simulink model "TestDrag"  (R2015a)
settings: Solver=ode45  StartTime=0.0  StopTime=inf  FixedStep=0.01  RelTol=1e-3
libraries: dspindex x9, simulink x7, dspnetwork x3, aerolibconvert2 x2, IMU_Library x1, GPS_Library x1, realtime_pacer_lib x1, etargetslib x1
settings Model: ParamWorkspaceSource=ReferencedWorkspace  CovSFcnEnable=off  Creator=abdkadma  LastModifiedBy=theth
settings OptimizationCC: InlineParams=on  InlineInvariantSignals=on  EnhancedBackFolding=on  ExpressionDepthLimit=2147483647  EfficientFloat2IntCast=on  SimCompilerOptimization=on
settings DebuggingCC: UnderspecifiedInitializationDetection=Classic  MergeDetectMultiDrivingBlocksExec=none  SolverPrmCheckMsg=warning  StateNameClashWarn=warning
settings RTWCC: RTWCompilerOptimization=on  CheckMdlBeforeBuild=Warning
settings GRTTargetCC: MatFileLogging=off  SupportNonFinite=off

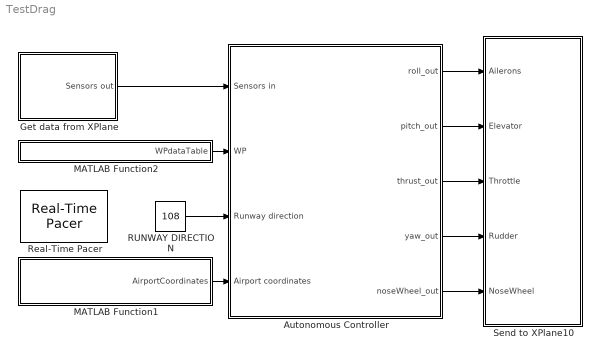
== system TestDrag ==
  "Autonomous Controller " : Subsystem
  Get data from XPlane : Subsystem  Description=|  TreatAsAtomicUnit=on  mask(Get Data from Xplane10){remoteURL='127.0.0.1', localPort=49005, sampletime=0.02}
      | Done by: Mohamed Abdelkader
      | Contact for updates: mohamedashraf123@gmail.com
      mask prompts: remoteURL "Remote IP address ('0.0.0.0' to accept all):(default='127.0.0.1')"; localPort "Local IP port: that Xplane10 sends to (default=49005)"; sampletime "Sampling time (seconds), how frequenlty to capture data from Xplane. Don't set to low as it might not be able to capture the smaples from Xplane. Default is 0.02 assuming the UDP rate in Xplane is set to 50 sample per second"
      mask help:
      | Get Data from X-Plane10
      | * make sure you configure the right port
      | and the right IP address
      mask TypeOptions remoteURL: UDP Receive1/remoteURL
      mask TypeOptions localPort: UDP Receive1/localPort
      mask TypeOptions sampletime: UDP Receive1/sampletime
  MATLAB Function1 : MATLAB Function  TreatAsAtomicUnit=on
  MATLAB Function2 : MATLAB Function  TreatAsAtomicUnit=on
  RUNWAY DIRECTION : Constant  Value=108
  Real-Time Pacer : realtime_pacer_lib/Real-Time Pacer  simTimePerRealTime=1
  Send to XPlane10 : Subsystem  Description=|  mask(Send Commands to X-Plane 10){remoteURL='127.0.0.1', remotePort=49000}
      | Done by: Mohamed Abdelkader
      | Contact for updates: mohamedashraf123@gmail.com
      mask prompts: remoteURL "Remote IP address (default='127.0.0.1'): X-Plane10 IP"; remotePort "Remote IP port:X-Plane10 port(default=49000)"
      mask help:
      | Sends Control Surfaces Commands to Xplane10
      | Throttle in [0,1]
      | Elevator, Ailerons, rudder, nosewheel in [-1,1]
      mask TypeOptions remoteURL: UDP Send/remoteURL
      mask TypeOptions remotePort: UDP Send/remotePort
  wires:
  "Autonomous Controller "/1(roll_out) -> Send to XPlane10/1(Ailerons)
  "Autonomous Controller "/2(pitch_out) -> Send to XPlane10/2(Elevator)
  "Autonomous Controller "/3(thrust_out) -> Send to XPlane10/3(Throttle)
  "Autonomous Controller "/4(yaw_out) -> Send to XPlane10/4(Rudder)
  "Autonomous Controller "/5(noseWheel_out) -> Send to XPlane10/5(NoseWheel)
  Get data from XPlane/1(Sensors out) -> "Autonomous Controller "/1(Sensors in)
  RUNWAY DIRECTION/1 -> "Autonomous Controller "/3(Runway direction)
  MATLAB Function1/1(AirportCoordinates) -> "Autonomous Controller "/4(Airport coordinates)
  MATLAB Function2/1(WPdataTable) -> "Autonomous Controller "/2(WP)

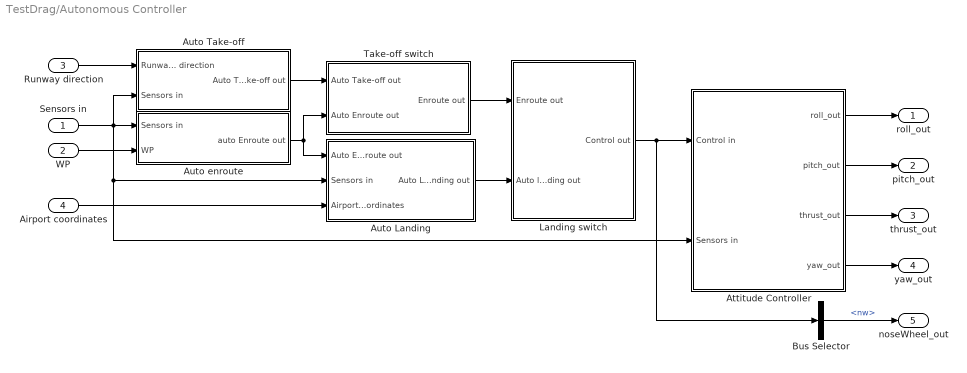
== system TestDrag/Autonomous Controller  ==
  Sensors in : Inport
  WP : Inport  Port=2
  Runway direction : Inport  Port=3
  Airport coordinates : Inport  Port=4
  Attitude Controller : Subsystem
  Auto Landing : Subsystem
  Auto Take-off : Subsystem
  Auto enroute : Subsystem
  Bus Selector : BusSelector  OutputSignals=nw
  Landing switch : Subsystem
  Take-off switch : Subsystem
  roll_out : Outport
  pitch_out : Outport  Port=2
  thrust_out : Outport  Port=3
  yaw_out : Outport  Port=4
  noseWheel_out : Outport  Port=5
  wires:
  Take-off switch/1(Enroute out) -> Landing switch/1(Enroute out)
  Auto Landing/1(Auto Landing out) -> Landing switch/2(Auto landing out)
  Auto enroute/1(auto Enroute out) -> Auto Landing/1(Auto Enroute out), Take-off switch/2(Auto Enroute out)
  Attitude Controller/4(yaw_out) -> yaw_out/1
  Attitude Controller/1(roll_out) -> roll_out/1
  Attitude Controller/3(thrust_out) -> thrust_out/1
  Auto Take-off/1(Auto Take-off out) -> Take-off switch/1(Auto Take-off out)
  Sensors in/1 -> Auto enroute/1(Sensors in), Auto Take-off/2(Sensors in), Attitude Controller/2(Sensors in), Auto Landing/2(Sensors in)
  Runway direction/1 -> Auto Take-off/1(Runway direction)
  Landing switch/1(Control out) -> Attitude Controller/1(Control in), Bus Selector/1
  Bus Selector/1 -> noseWheel_out/1  "<nw>"
  Attitude Controller/2(pitch_out) -> pitch_out/1
  Airport coordinates/1 -> Auto Landing/3(Airport coordinates)
  WP/1 -> Auto enroute/2(WP)

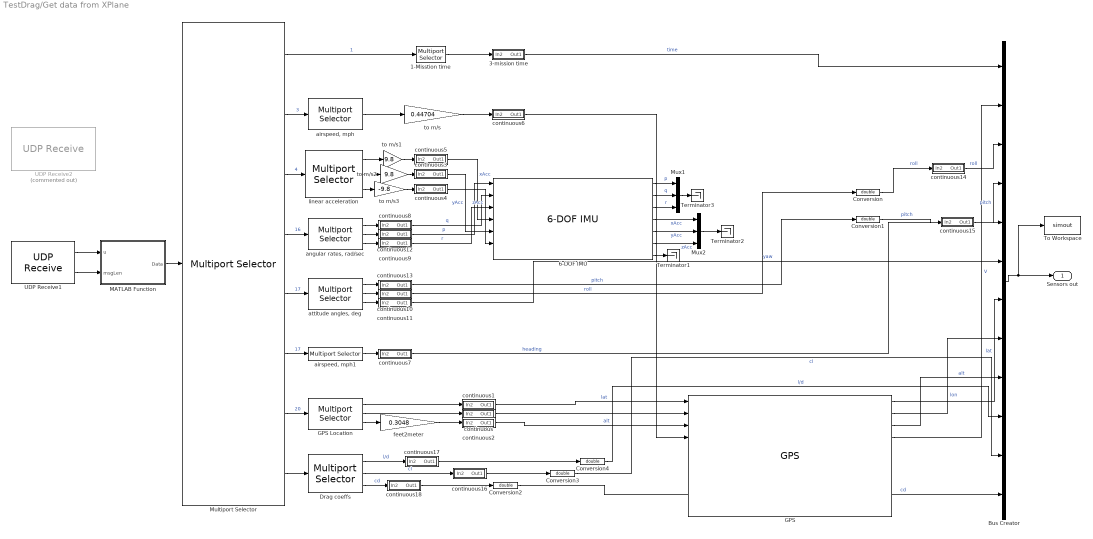
== system TestDrag/Get data from XPlane ==
  1-Misstion time : dspindex/Multiport Selector  rowsOrCols=Columns  idxCellArray={3}  idxErrMode=Clip Index
  3-mission time : Subsystem
  6-DOF IMU : IMU_Library/6-DOF IMU  lpf_filt_freq_hz_ix=20 Hz  gyro_scale_ix=+/- 500 deg/sec  accel_scale_ix=+/- 8g  SampleTime=0.02  lpf_filt_freq_hz=5 Hz  gyro_scale=+/- 250 deg/sec  accel_scale=+/- 2g
  Bus Creator : BusCreator  Inputs='time','V','roll','pitch','heading','yaw','lat','lon','alt','l/d','cl','cd'
  Conversion{,1..4} (5 alike) : DataTypeConversion  OutDataTypeStr=double
  Drag coeffs : dspindex/Multiport Selector  rowsOrCols=Columns  idxCellArray={1,3,4}  idxErrMode=Clip Index
  GPS : GPS_Library/GPS
  GPS Location : dspindex/Multiport Selector  rowsOrCols=Columns  idxCellArray={1,2,3}  idxErrMode=Clip Index
  MATLAB Function : MATLAB Function  TreatAsAtomicUnit=on
  Multiport Selector : dspindex/Multiport Selector  rowsOrCols=Rows  idxCellArray={1,3,4,16,17,18,20,68}  idxErrMode=Clip Index
  Mux1 : Mux  Inputs=3
  Mux2 : Mux  Inputs=3
  Terminator1 : Terminator
  Terminator2 : Terminator
  Terminator3 : Terminator
  To Workspace : ToWorkspace  VariableName=simout  SampleTime=-1
      settings: Save2DSignal=2-D array (concatenate along first dimension)
  UDP Receive1 : dspnetwork/UDP Receive  localURL='0.0.0.0'  localPort=localPort  remoteURL=remoteURL  remotePort=-1  recvBufferSize=8192  dims=365*20  signalDatatype=uint8  isVarSize=off  showBlockingTime=off  blockingTime=0  sampletime=sampletime
  UDP Receive2 : dspnetwork/UDP Receive  Commented=on  localURL='0.0.0.0'  localPort=localPort  remoteURL=remoteURL  remotePort=-1  recvBufferSize=8192  dims=365  signalDatatype=uint8  isVarSize=off  showBlockingTime=on  blockingTime=0.01  sampletime=0.01  blockPlatform=LINUX
  "airspeed, mph" : dspindex/Multiport Selector  rowsOrCols=Columns  idxCellArray={6}  idxErrMode=Clip Index
  "airspeed, mph1" : dspindex/Multiport Selector  rowsOrCols=Columns  idxCellArray={3}  idxErrMode=Clip Index
  "angular rates, rad/sec" : dspindex/Multiport Selector  rowsOrCols=Columns  idxCellArray={1,2,3}  idxErrMode=Clip Index
  "attitude angles, deg" : dspindex/Multiport Selector  rowsOrCols=Columns  idxCellArray={1,2,3}  idxErrMode=Clip Index
  continuous : Subsystem
  continuous1 : Subsystem
  continuous10 : Subsystem
  continuous11 : Subsystem
  continuous12 : Subsystem
  continuous13 : Subsystem
  continuous14 : Subsystem
  continuous15 : Subsystem
  continuous16 : Subsystem
  continuous17 : Subsystem
  continuous18 : Subsystem
  continuous2 : Subsystem
  continuous3 : Subsystem
  continuous4 : Subsystem
  continuous5 : Subsystem
  continuous6 : Subsystem
  continuous7 : Subsystem
  continuous8 : Subsystem
  continuous9 : Subsystem
  feet2meter : Gain  Gain=0.3048
  linear acceleration : dspindex/Multiport Selector  rowsOrCols=Columns  idxCellArray={6,7,5}  idxErrMode=Clip Index
  to m/s : Gain  Gain=0.44704
  to m/s1 : Gain  Gain=9.8
  to m/s2 : Gain  Gain=9.8
  to m/s3 : Gain  Gain=-9.8
  Sensors out : Outport
  wires:
  "attitude angles, deg"/3 -> continuous11/1(In2)
  "angular rates, rad/sec"/3 -> continuous9/1(In2)
  MATLAB Function/1(Data) -> Multiport Selector/1
  linear acceleration/2 -> to m/s2/1
  to m/s2/1 -> continuous3/1(In2)
  to m/s1/1 -> continuous5/1(In2)
  "attitude angles, deg"/1 -> continuous13/1(In2)
  "attitude angles, deg"/2 -> continuous10/1(In2)
  to m/s/1 -> continuous6/1(In2)
  "airspeed, mph"/1 -> to m/s/1
  linear acceleration/1 -> to m/s1/1
  "angular rates, rad/sec"/1 -> continuous8/1(In2)
  linear acceleration/3 -> to m/s3/1
  "angular rates, rad/sec"/2 -> continuous12/1(In2)
  "airspeed, mph1"/1 -> continuous7/1(In2)
  to m/s3/1 -> continuous4/1(In2)
  feet2meter/1 -> continuous2/1(In2)
  UDP Receive1/1 -> MATLAB Function/1(u)
  UDP Receive1/2 -> MATLAB Function/2(msgLen)
  GPS Location/3 -> feet2meter/1
  GPS Location/2 -> continuous/1(In2)
  GPS Location/1 -> continuous1/1(In2)
  continuous11/1(Out1) -> Bus Creator/6  "yaw"
  Bus Creator/1 -> To Workspace/1, Sensors out/1
  Multiport Selector/4 -> "angular rates, rad/sec"/1  "16"
  Multiport Selector/5 -> "attitude angles, deg"/1  "17"
  Multiport Selector/6 -> "airspeed, mph1"/1  "17"
  Multiport Selector/7 -> GPS Location/1  "20"
  1-Misstion time/1 -> 3-mission time/1(In2)
  Multiport Selector/1 -> 1-Misstion time/1  "1"
  Multiport Selector/2 -> "airspeed, mph"/1  "3"
  Multiport Selector/3 -> linear acceleration/1  "4"
  continuous5/1(Out1) -> 6-DOF IMU/4  "xAcc"
  continuous3/1(Out1) -> 6-DOF IMU/5  "yAcc"
  continuous4/1(Out1) -> 6-DOF IMU/6  "zAcc"
  continuous12/1(Out1) -> 6-DOF IMU/1  "p"
  continuous8/1(Out1) -> 6-DOF IMU/2  "q"
  continuous9/1(Out1) -> 6-DOF IMU/3  "r"
  continuous1/1(Out1) -> GPS/1  "lat"
  GPS/1 -> Bus Creator/7  "lat"
  continuous/1(Out1) -> GPS/2
  GPS/2 -> Bus Creator/8  "lon"
  continuous2/1(Out1) -> GPS/3  "alt"
  GPS/3 -> Bus Creator/9  "alt"
  continuous6/1(Out1) -> GPS/4
  GPS/4 -> Bus Creator/2  "V"
  continuous7/1(Out1) -> Bus Creator/5  "heading"
  3-mission time/1(Out1) -> Bus Creator/1  "time"
  6-DOF IMU/7 -> Terminator1/1
  6-DOF IMU/1 -> Mux1/1  "p"
  6-DOF IMU/2 -> Mux1/2  "q"
  6-DOF IMU/3 -> Mux1/3  "r"
  6-DOF IMU/4 -> Mux2/1  "xAcc"
  6-DOF IMU/5 -> Mux2/2  "yAcc"
  6-DOF IMU/6 -> Mux2/3  "zAcc"
  continuous13/1(Out1) -> Conversion1/1  "pitch"
  continuous10/1(Out1) -> Conversion/1  "roll"
  Conversion/1 -> continuous14/1(In2)  "roll"
  Conversion1/1 -> continuous15/1(In2)  "pitch"
  continuous14/1(Out1) -> Bus Creator/3  "roll"
  continuous15/1(Out1) -> Bus Creator/4  "pitch"
  Mux1/1 -> Terminator3/1
  Mux2/1 -> Terminator2/1
  Multiport Selector/8 -> Drag coeffs/1
  Drag coeffs/1 -> continuous17/1(In2)  "l/d"
  Drag coeffs/2 -> continuous16/1(In2)  "cl"
  Drag coeffs/3 -> continuous18/1(In2)  "cd"
  Conversion2/1 -> Bus Creator/12  "cd"
  Conversion3/1 -> Bus Creator/11  "cl"
  Conversion4/1 -> Bus Creator/10  "l/d"
  continuous17/1(Out1) -> Conversion4/1
  continuous16/1(Out1) -> Conversion3/1
  continuous18/1(Out1) -> Conversion2/1

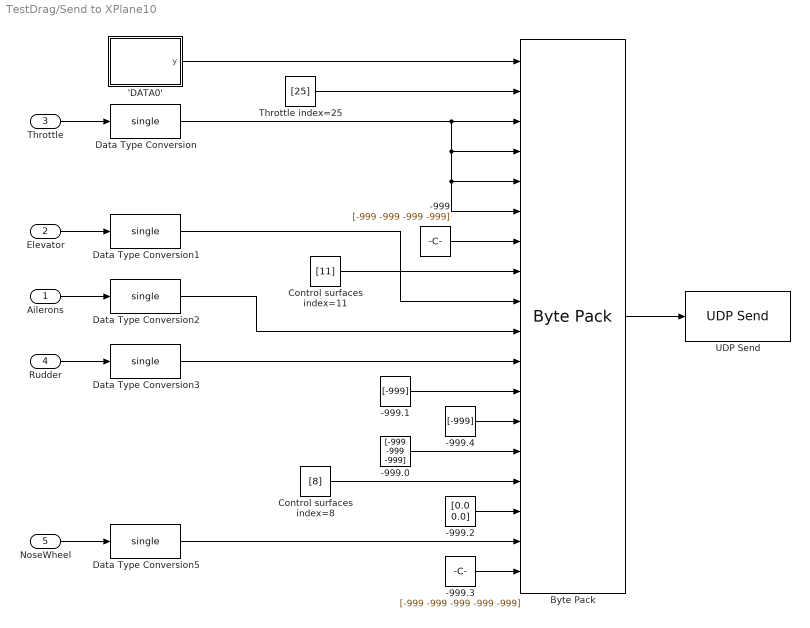
== system TestDrag/Send to XPlane10 ==
  Ailerons : Inport
  Elevator : Inport  Port=2
  Throttle : Inport  Port=3
  Rudder : Inport  Port=4
  NoseWheel : Inport  Port=5
  'DATA0' : MATLAB Function  TreatAsAtomicUnit=on
  -999 : Constant  Value=[-999 -999 -999 -999]  OutDataTypeStr=int32  SampleTime=-1
  -999.0 : Constant  Value=[-999 -999 -999]  OutDataTypeStr=int32  SampleTime=-1
  -999.1 : Constant  Value=[-999]  OutDataTypeStr=int32  SampleTime=-1
  -999.2 : Constant  Value=[0.0 0.0]  OutDataTypeStr=single  SampleTime=-1
  -999.3 : Constant  Value=[-999 -999 -999 -999 -999]  OutDataTypeStr=int32  SampleTime=-1
  -999.4 : Constant  Value=[-999]  OutDataTypeStr=single  SampleTime=-1
  Byte Pack : etargetslib/Byte Pack  datatypes={'uint8','uint32','single','single','single','single','int32','uint32','single','single','single','int32','single','int32','uint32','single','single','int32'}  byteAlign=1
  Control surfaces index=11 : Constant  Value=[11]  OutDataTypeStr=uint32  SampleTime=-1
  Control surfaces index=8 : Constant  Value=[8]  OutDataTypeStr=uint32  SampleTime=-1
  Data Type Conversion : DataTypeConversion  OutMin=[0]  OutMax=[1.0]  OutDataTypeStr=single
  Data Type Conversion{1..3,5} (4 alike) : DataTypeConversion  OutMin=[-1.0]  OutMax=[1.0]  OutDataTypeStr=single
  Throttle index=25 : Constant  Value=[25]  OutDataTypeStr=uint32  SampleTime=-1
  UDP Send : dspnetwork/UDP Send  remoteURL=remoteURL  remotePort=remotePort  localURL='0.0.0.0'  localPortSource=Automatically determine  localPort=-1  sampletime=-1  separateLengthPort=0
  wires:
  Ailerons/1 -> Data Type Conversion2/1
  Control surfaces index=11/1 -> Byte Pack/8
  Throttle/1 -> Data Type Conversion/1
  Data Type Conversion1/1 -> Byte Pack/9
  'DATA0'/1(y) -> Byte Pack/1
  Throttle index=25/1 -> Byte Pack/2
  Byte Pack/1 -> UDP Send/1
  -999/1 -> Byte Pack/7
  Data Type Conversion2/1 -> Byte Pack/10
  Data Type Conversion3/1 -> Byte Pack/11
  Rudder/1 -> Data Type Conversion3/1
  -999.0/1 -> Byte Pack/14
  Elevator/1 -> Data Type Conversion1/1
  Data Type Conversion/1 -> Byte Pack/3, Byte Pack/4, Byte Pack/6, Byte Pack/5
  -999.1/1 -> Byte Pack/12
  Control surfaces index=8/1 -> Byte Pack/15
  -999.2/1 -> Byte Pack/16
  Data Type Conversion5/1 -> Byte Pack/17
  NoseWheel/1 -> Data Type Conversion5/1
  -999.3/1 -> Byte Pack/18
  -999.4/1 -> Byte Pack/13

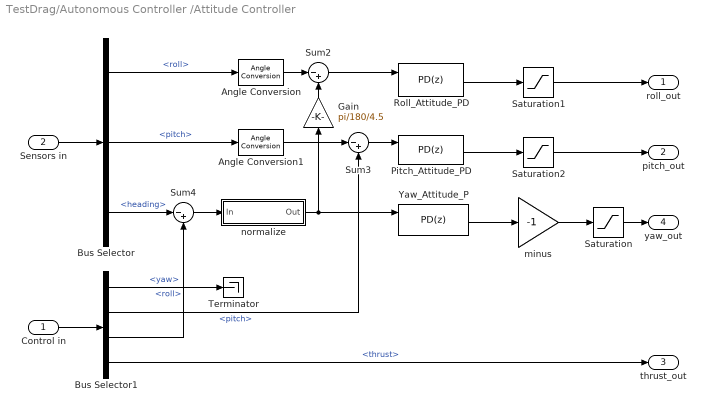
== system TestDrag/Autonomous Controller /Attitude Controller ==
  Control in : Inport
  Sensors in : Inport  Port=2
  Angle Conversion : aerolibconvert2/Angle Conversion  IU=deg  OU=rad
  Angle Conversion1 : aerolibconvert2/Angle Conversion  IU=deg  OU=rad
  Bus Selector : BusSelector  OutputSignals=roll,pitch,heading
  Bus Selector1 : BusSelector  OutputSignals=roll,pitch,yaw,thrust
  Gain : Gain  Gain=pi/180/4.5
  Pitch_Attitude_PD : simulink/Continuous/PID Controller  Controller=PD  TimeDomain=Discrete-time  SampleTime=0.02  IntegratorMethod=Forward Euler  FilterMethod=Forward Euler  Form=Parallel  UseFilter=off  ControllerParametersSource=internal  P=1  I=0  D=0.04  N=20  InitialConditionSource=internal  InitialConditionForIntegrator=0  InitialConditionForFilter=0  ExternalReset=either  LimitOutput=on  UpperSaturationLimit=1  LowerSaturationLimit=-1  LinearizeAsGain=on  AntiWindupMode=none  Kb=1  TrackingMode=off  Kt=1  PParamMin=[]  PParamMax=[]  IParamMin=[]  IParamMax=[]  DParamMin=[]  DParamMax=[]  NParamMin=[]  NParamMax=[]  KbParamMin=[]  KbParamMax=[]  KtParamMin=[]  KtParamMax=[]  POutMin=[]  POutMax=[]  IOutMin=[]  IOutMax=[]  DOutMin=[]  DOutMax=[]  NOutMin=[]  NOutMax=[]  KbOutMin=[]  KbOutMax=[]  KtOutMin=[]  KtOutMax=[]  IntegratorOutMin=[]  IntegratorOutMax=[]  FilterOutMin=[]  FilterOutMax=[]  SumOutMin=[]  SumOutMax=[]  SumI1OutMin=[]  SumI1OutMax=[]  SumI2OutMin=[]  SumI2OutMax=[]  SumI3OutMin=[]  SumI3OutMax=[]  SumDOutMin=[]  SumDOutMax=[]  SaturationOutMin=[]  SaturationOutMax=[]  IntegratorContinuousStateAttributes=''  IntegratorStateMustResolveToSignalObject=off  IntegratorRTWStateStorageClass=Auto  FilterContinuousStateAttributes=''  FilterStateMustResolveToSignalObject=off  FilterRTWStateStorageClass=Auto  DifferentiatorICPrevScaledInput=0  DifferentiatorOutMin=[]  DifferentiatorOutMax=[]
  Roll_Attitude_PD : simulink/Continuous/PID Controller  Controller=PD  TimeDomain=Discrete-time  SampleTime=0.02  IntegratorMethod=Forward Euler  FilterMethod=Forward Euler  Form=Parallel  UseFilter=off  ControllerParametersSource=internal  P=1  I=0  D=0.0008  N=20  InitialConditionSource=internal  InitialConditionForIntegrator=0  InitialConditionForFilter=0  ExternalReset=either  LimitOutput=on  UpperSaturationLimit=1  LowerSaturationLimit=-1  LinearizeAsGain=on  AntiWindupMode=none  Kb=1  TrackingMode=off  Kt=1  PParamMin=[]  PParamMax=[]  IParamMin=[]  IParamMax=[]  DParamMin=[]  DParamMax=[]  NParamMin=[]  NParamMax=[]  KbParamMin=[]  KbParamMax=[]  KtParamMin=[]  KtParamMax=[]  POutMin=[]  POutMax=[]  IOutMin=[]  IOutMax=[]  DOutMin=[]  DOutMax=[]  NOutMin=[]  NOutMax=[]  KbOutMin=[]  KbOutMax=[]  KtOutMin=[]  KtOutMax=[]  IntegratorOutMin=[]  IntegratorOutMax=[]  FilterOutMin=[]  FilterOutMax=[]  SumOutMin=[]  SumOutMax=[]  SumI1OutMin=[]  SumI1OutMax=[]  SumI2OutMin=[]  SumI2OutMax=[]  SumI3OutMin=[]  SumI3OutMax=[]  SumDOutMin=[]  SumDOutMax=[]  SaturationOutMin=[]  SaturationOutMax=[]  IntegratorContinuousStateAttributes=''  IntegratorStateMustResolveToSignalObject=off  IntegratorRTWStateStorageClass=Auto  FilterContinuousStateAttributes=''  FilterStateMustResolveToSignalObject=off  FilterRTWStateStorageClass=Auto  DifferentiatorICPrevScaledInput=0  DifferentiatorOutMin=[]  DifferentiatorOutMax=[]
  Saturation : Saturate  UpperLimit=1  LowerLimit=-1
  Saturation1 : Saturate  UpperLimit=0.05  LowerLimit=-0.05
  Saturation2 : Saturate  UpperLimit=1  LowerLimit=-1
  Sum2 : Sum  Inputs=|-+
  Sum3 : Sum  Inputs=|-+
  Sum4 : Sum  Inputs=|-+
  Terminator : Terminator
  Yaw_Attitude_P : simulink/Continuous/PID Controller  Controller=PD  TimeDomain=Discrete-time  SampleTime=0.02  IntegratorMethod=Forward Euler  FilterMethod=Forward Euler  Form=Parallel  UseFilter=off  ControllerParametersSource=internal  P=pi/180  I=0  D=0.000034  N=100  InitialConditionSource=internal  InitialConditionForIntegrator=0  InitialConditionForFilter=0  ExternalReset=either  LimitOutput=on  UpperSaturationLimit=1  LowerSaturationLimit=-1  LinearizeAsGain=on  AntiWindupMode=none  Kb=1  TrackingMode=off  Kt=1  PParamMin=[]  PParamMax=[]  IParamMin=[]  IParamMax=[]  DParamMin=[]  DParamMax=[]  NParamMin=[]  NParamMax=[]  KbParamMin=[]  KbParamMax=[]  KtParamMin=[]  KtParamMax=[]  POutMin=[]  POutMax=[]  IOutMin=[]  IOutMax=[]  DOutMin=[]  DOutMax=[]  NOutMin=[]  NOutMax=[]  KbOutMin=[]  KbOutMax=[]  KtOutMin=[]  KtOutMax=[]  IntegratorOutMin=[]  IntegratorOutMax=[]  FilterOutMin=[]  FilterOutMax=[]  SumOutMin=[]  SumOutMax=[]  SumI1OutMin=[]  SumI1OutMax=[]  SumI2OutMin=[]  SumI2OutMax=[]  SumI3OutMin=[]  SumI3OutMax=[]  SumDOutMin=[]  SumDOutMax=[]  SaturationOutMin=[]  SaturationOutMax=[]  IntegratorContinuousStateAttributes=''  IntegratorStateMustResolveToSignalObject=off  IntegratorRTWStateStorageClass=Auto  FilterContinuousStateAttributes=''  FilterStateMustResolveToSignalObject=off  FilterRTWStateStorageClass=Auto  DifferentiatorICPrevScaledInput=0  DifferentiatorOutMin=[]  DifferentiatorOutMax=[]
  minus : Gain  Gain=-1
  normalize : Subsystem
  roll_out : Outport
  pitch_out : Outport  Port=2
  thrust_out : Outport  Port=3
  yaw_out : Outport  Port=4
  wires:
  Sum2/1 -> Roll_Attitude_PD/1
  Sum3/1 -> Pitch_Attitude_PD/1
  Angle Conversion/1 -> Sum2/1
  Angle Conversion1/1 -> Sum3/1
  Bus Selector/1 -> Angle Conversion/1  "<roll>"
  Bus Selector/2 -> Angle Conversion1/1  "<pitch>"
  minus/1 -> Saturation/1
  Bus Selector/3 -> Sum4/1  "<heading>"
  Sum4/1 -> normalize/1(In)
  normalize/1(Out) -> Gain/1, Yaw_Attitude_P/1
  Sensors in/1 -> Bus Selector/1
  Control in/1 -> Bus Selector1/1
  Bus Selector1/2 -> Sum3/2  "<pitch>"
  Bus Selector1/4 -> thrust_out/1  "<thrust>"
  Bus Selector1/3 -> Sum4/2  "<yaw>"
  Gain/1 -> Sum2/2
  Saturation1/1 -> roll_out/1
  Saturation2/1 -> pitch_out/1
  Yaw_Attitude_P/1 -> minus/1
  Pitch_Attitude_PD/1 -> Saturation2/1
  Roll_Attitude_PD/1 -> Saturation1/1
  Saturation/1 -> yaw_out/1
  Bus Selector1/1 -> Terminator/1  "<roll>"

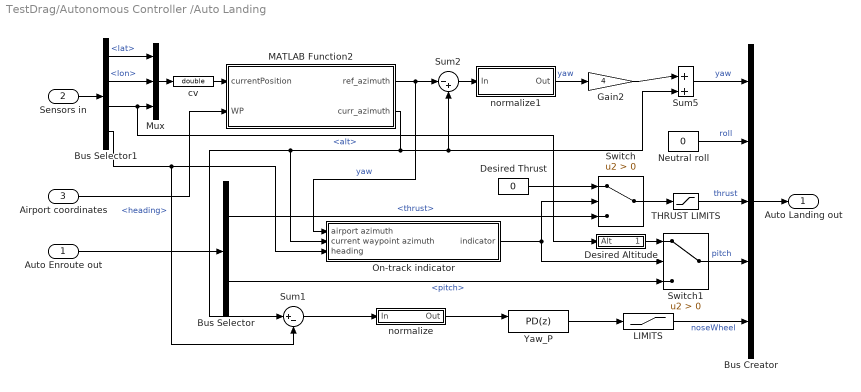
== system TestDrag/Autonomous Controller /Auto Landing ==
  Auto Enroute out : Inport
  Sensors in : Inport  Port=2
  Airport coordinates : Inport  Port=3
  Bus Creator : BusCreator  Inputs='yaw','roll','thrust','pitch','noseWheel'
  Bus Selector : BusSelector  OutputSignals=thrust,pitch
  Bus Selector1 : BusSelector  OutputSignals=lat,lon,alt,heading
  Desired Altitude : Subsystem
  Desired Thrust : Constant  Value=0  OutDataTypeStr=single
  Gain2 : Gain  Gain=4
  LIMITS : Saturate
  MATLAB Function2 : MATLAB Function  TreatAsAtomicUnit=on
  Mux : Mux  Inputs=3
  Neutral roll : Constant  Value=0  OutDataTypeStr=single
  On-track indicator : Subsystem
  Sum1 : Sum  Inputs=|+-
  Sum2 : Sum  Inputs=|-+
  Sum5 : Sum  Inputs=|++
  Switch : Switch  Criteria=u2 > Threshold
  Switch1 : Switch  Criteria=u2 > Threshold
  THRUST LIMITS : Saturate  UpperLimit=1  LowerLimit=0
  Yaw_P : simulink/Continuous/PID Controller  Controller=PD  TimeDomain=Discrete-time  SampleTime=0.05  IntegratorMethod=Forward Euler  FilterMethod=Forward Euler  Form=Parallel  UseFilter=off  ControllerParametersSource=internal  P=0.016  I=0  D=0.0024  N=100  InitialConditionSource=internal  InitialConditionForIntegrator=0  InitialConditionForFilter=0  ExternalReset=either  LimitOutput=on  UpperSaturationLimit=1  LowerSaturationLimit=-1  LinearizeAsGain=on  AntiWindupMode=none  Kb=1  TrackingMode=off  Kt=1  PParamMin=[]  PParamMax=[]  IParamMin=[]  IParamMax=[]  DParamMin=[]  DParamMax=[]  NParamMin=[]  NParamMax=[]  KbParamMin=[]  KbParamMax=[]  KtParamMin=[]  KtParamMax=[]  POutMin=[]  POutMax=[]  IOutMin=[]  IOutMax=[]  DOutMin=[]  DOutMax=[]  NOutMin=[]  NOutMax=[]  KbOutMin=[]  KbOutMax=[]  KtOutMin=[]  KtOutMax=[]  IntegratorOutMin=[]  IntegratorOutMax=[]  FilterOutMin=[]  FilterOutMax=[]  SumOutMin=[]  SumOutMax=[]  SumI1OutMin=[]  SumI1OutMax=[]  SumI2OutMin=[]  SumI2OutMax=[]  SumI3OutMin=[]  SumI3OutMax=[]  SumDOutMin=[]  SumDOutMax=[]  SaturationOutMin=[]  SaturationOutMax=[]  IntegratorContinuousStateAttributes=''  IntegratorStateMustResolveToSignalObject=off  IntegratorRTWStateStorageClass=Auto  FilterContinuousStateAttributes=''  FilterStateMustResolveToSignalObject=off  FilterRTWStateStorageClass=Auto  DifferentiatorICPrevScaledInput=0  DifferentiatorOutMin=[]  DifferentiatorOutMax=[]
  cv : DataTypeConversion  OutDataTypeStr=double
  normalize : Subsystem
  normalize1 : Subsystem
  Auto Landing out : Outport
  wires:
  THRUST LIMITS/1 -> Bus Creator/3  "thrust"
  Airport coordinates/1 -> MATLAB Function2/2(WP)
  MATLAB Function2/2(curr_azimuth) -> Sum1/1, On-track indicator/2(current waypoint azimuth), Sum5/2, Sum2/2
  LIMITS/1 -> Bus Creator/5  "noseWheel"
  MATLAB Function2/1(ref_azimuth) -> Sum2/1, On-track indicator/1(airport azimuth)  "yaw"
  normalize/1(Out) -> Yaw_P/1
  Auto Enroute out/1 -> Bus Selector/1
  Bus Selector/1 -> Switch/3  "<thrust>"
  Neutral roll/1 -> Bus Creator/2  "roll"
  Sum1/1 -> normalize/1(In)
  Bus Creator/1 -> Auto Landing out/1
  Sensors in/1 -> Bus Selector1/1
  Bus Selector1/1 -> Mux/1  "<lat>"
  Bus Selector1/2 -> Mux/2  "<lon>"
  Bus Selector1/3 -> Desired Altitude/1(Alt), Mux/3  "<alt>"
  Sum2/1 -> normalize1/1(In)
  Bus Selector1/4 -> Sum1/2, On-track indicator/3(heading)  "<heading>"
  Desired Thrust/1 -> Switch/1
  Bus Selector/2 -> Switch1/3  "<pitch>"
  Switch/1 -> THRUST LIMITS/1
  Switch1/1 -> Bus Creator/4  "pitch"
  normalize1/1(Out) -> Gain2/1  "yaw"
  Sum5/1 -> Bus Creator/1  "yaw"
  On-track indicator/1(indicator) -> Switch1/2, Switch/2
  Gain2/1 -> Sum5/1
  Mux/1 -> cv/1
  cv/1 -> MATLAB Function2/1(currentPosition)
  Yaw_P/1 -> LIMITS/1
  Desired Altitude/1(pitch) -> Switch1/1

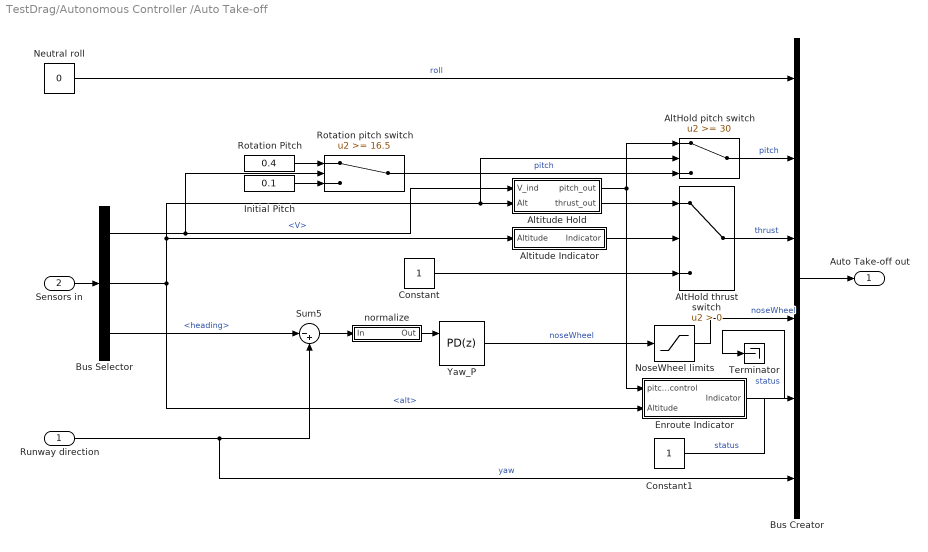
== system TestDrag/Autonomous Controller /Auto Take-off ==
  Runway direction : Inport
  Sensors in : Inport  Port=2
  AltHold pitch switch : Switch  Threshold=30
  AltHold thrust switch : Switch  Criteria=u2 > Threshold
  Altitude Hold : Subsystem
  Altitude Indicator : Subsystem
  Bus Creator : BusCreator  Inputs='roll','pitch','thrust','noseWheel','status','yaw'
  Bus Selector : BusSelector  OutputSignals=V,alt,heading
  Constant : Constant
  Constant1 : Constant
  Enroute Indicator : Subsystem
  Initial Pitch : Constant  Value=0.1  OutDataTypeStr=single
  Neutral roll : Constant  Value=0  OutDataTypeStr=single
  NoseWheel limits : Saturate
  Rotation Pitch : Constant  Value=0.4  OutDataTypeStr=single
  Rotation pitch switch : Switch  Threshold=16.5
  Sum5 : Sum  Inputs=|-+
  Terminator : Terminator
  Yaw_P : simulink/Continuous/PID Controller  Controller=PD  TimeDomain=Discrete-time  SampleTime=0.02  IntegratorMethod=Forward Euler  FilterMethod=Forward Euler  Form=Parallel  UseFilter=off  ControllerParametersSource=internal  P=0.012  I=0  D=0.0024  N=100  InitialConditionSource=internal  InitialConditionForIntegrator=0  InitialConditionForFilter=0  ExternalReset=either  LimitOutput=on  UpperSaturationLimit=1  LowerSaturationLimit=-1  LinearizeAsGain=on  AntiWindupMode=none  Kb=1  TrackingMode=off  Kt=1  PParamMin=[]  PParamMax=[]  IParamMin=[]  IParamMax=[]  DParamMin=[]  DParamMax=[]  NParamMin=[]  NParamMax=[]  KbParamMin=[]  KbParamMax=[]  KtParamMin=[]  KtParamMax=[]  POutMin=[]  POutMax=[]  IOutMin=[]  IOutMax=[]  DOutMin=[]  DOutMax=[]  NOutMin=[]  NOutMax=[]  KbOutMin=[]  KbOutMax=[]  KtOutMin=[]  KtOutMax=[]  IntegratorOutMin=[]  IntegratorOutMax=[]  FilterOutMin=[]  FilterOutMax=[]  SumOutMin=[]  SumOutMax=[]  SumI1OutMin=[]  SumI1OutMax=[]  SumI2OutMin=[]  SumI2OutMax=[]  SumI3OutMin=[]  SumI3OutMax=[]  SumDOutMin=[]  SumDOutMax=[]  SaturationOutMin=[]  SaturationOutMax=[]  IntegratorContinuousStateAttributes=''  IntegratorStateMustResolveToSignalObject=off  IntegratorRTWStateStorageClass=Auto  FilterContinuousStateAttributes=''  FilterStateMustResolveToSignalObject=off  FilterRTWStateStorageClass=Auto  DifferentiatorICPrevScaledInput=0  DifferentiatorOutMin=[]  DifferentiatorOutMax=[]
  normalize : Subsystem
  Auto Take-off out : Outport
  wires:
  Rotation Pitch/1 -> Rotation pitch switch/1
  Initial Pitch/1 -> Rotation pitch switch/3
  Neutral roll/1 -> Bus Creator/1  "roll"
  Bus Selector/3 -> Sum5/1  "<heading>"
  Runway direction/1 -> Sum5/2, Bus Creator/6  "yaw"
  Bus Selector/2 -> Altitude Indicator/1(Altitude), Altitude Hold/2(Alt), AltHold pitch switch/2, Enroute Indicator/2(Altitude)  "<alt>"
  Bus Selector/1 -> Rotation pitch switch/2, Altitude Hold/1(V_ind)  "<V>"
  Sum5/1 -> normalize/1(In)
  normalize/1(Out) -> Yaw_P/1
  Bus Creator/1 -> Auto Take-off out/1
  Sensors in/1 -> Bus Selector/1
  AltHold pitch switch/1 -> Bus Creator/2  "pitch"
  Rotation pitch switch/1 -> AltHold pitch switch/3  "pitch"
  AltHold thrust switch/1 -> Bus Creator/3  "thrust"
  Altitude Hold/2(thrust_out) -> AltHold thrust switch/1
  Altitude Hold/1(pitch_out) -> Enroute Indicator/1(pitch control), AltHold pitch switch/1
  Altitude Indicator/1(Indicator) -> AltHold thrust switch/2
  Yaw_P/1 -> NoseWheel limits/1  "noseWheel"
  Constant/1 -> AltHold thrust switch/3
  NoseWheel limits/1 -> Bus Creator/4  "noseWheel"
  Enroute Indicator/1(Indicator) -> Terminator/1  "status"
  Constant1/1 -> Bus Creator/5  "status"

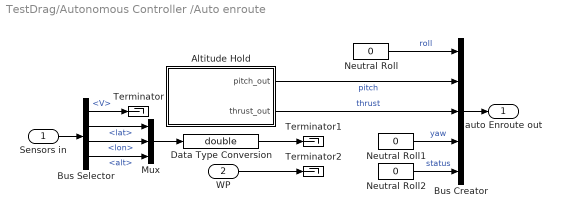
== system TestDrag/Autonomous Controller /Auto enroute ==
  Sensors in : Inport
  WP : Inport  Port=2
  Altitude Hold : Subsystem
  Bus Creator : BusCreator  Inputs='roll','pitch','thrust','yaw','status'
  Bus Selector : BusSelector  OutputSignals=V,lat,lon,alt
  Data Type Conversion : DataTypeConversion  OutDataTypeStr=double
  Mux : Mux  Inputs=3
  Neutral Roll : Constant  Value=0
  Neutral Roll1 : Constant  Value=0
  Neutral Roll2 : Constant  Value=0
  Terminator : Terminator
  Terminator1 : Terminator
  Terminator2 : Terminator
  auto Enroute out : Outport
  wires:
  WP/1 -> Terminator2/1
  Neutral Roll1/1 -> Bus Creator/4  "yaw"
  Neutral Roll2/1 -> Bus Creator/5  "status"
  Neutral Roll/1 -> Bus Creator/1  "roll"
  Bus Creator/1 -> auto Enroute out/1
  Altitude Hold/1(pitch_out) -> Bus Creator/2  "pitch"
  Altitude Hold/2(thrust_out) -> Bus Creator/3  "thrust"
  Sensors in/1 -> Bus Selector/1
  Bus Selector/2 -> Mux/1  "<lat>"
  Bus Selector/3 -> Mux/2  "<lon>"
  Bus Selector/4 -> Mux/3  "<alt>"
  Mux/1 -> Data Type Conversion/1
  Data Type Conversion/1 -> Terminator1/1
  Bus Selector/1 -> Terminator/1  "<V>"

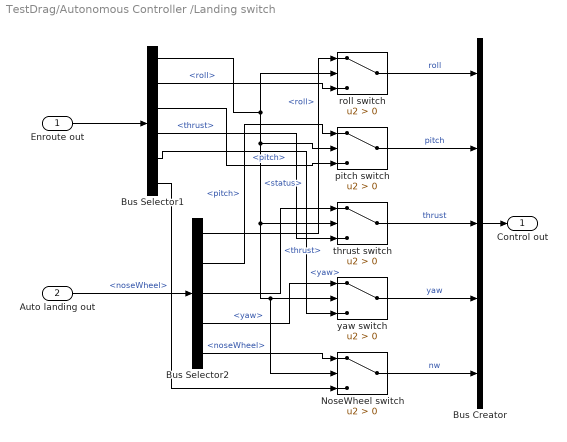
== system TestDrag/Autonomous Controller /Landing switch ==
  Enroute out : Inport
  Auto landing out : Inport  Port=2
  Bus Creator : BusCreator  Inputs='roll','pitch','thrust','yaw','nw'
  Bus Selector1 : BusSelector  OutputSignals=status,roll,pitch,thrust,yaw,noseWheel
  Bus Selector2 : BusSelector  OutputSignals=roll,pitch,thrust,yaw,noseWheel
  NoseWheel switch : Switch  Criteria=u2 > Threshold
  pitch switch : Switch  Criteria=u2 > Threshold
  roll switch : Switch  Criteria=u2 > Threshold
  thrust switch : Switch  Criteria=u2 > Threshold
  yaw switch : Switch  Criteria=u2 > Threshold
  Control out : Outport
  wires:
  Bus Selector1/2 -> roll switch/3  "<roll>"
  roll switch/1 -> Bus Creator/1  "roll"
  Bus Selector2/1 -> roll switch/1  "<roll>"
  Bus Selector1/3 -> pitch switch/3  "<pitch>"
  pitch switch/1 -> Bus Creator/2  "pitch"
  Bus Selector2/2 -> pitch switch/1  "<pitch>"
  Bus Selector1/4 -> thrust switch/3  "<thrust>"
  thrust switch/1 -> Bus Creator/3  "thrust"
  Bus Selector2/3 -> thrust switch/1  "<thrust>"
  Bus Selector1/5 -> yaw switch/3  "<yaw>"
  yaw switch/1 -> Bus Creator/4  "yaw"
  Bus Selector2/4 -> yaw switch/1  "<yaw>"
  Bus Selector1/1 -> roll switch/2, NoseWheel switch/2, yaw switch/2, thrust switch/2, pitch switch/2  "<status>"
  Bus Selector1/6 -> NoseWheel switch/3  "<noseWheel>"
  Bus Selector2/5 -> NoseWheel switch/1  "<noseWheel>"
  Enroute out/1 -> Bus Selector1/1
  Auto landing out/1 -> Bus Selector2/1
  Bus Creator/1 -> Control out/1
  NoseWheel switch/1 -> Bus Creator/5  "nw"

== system TestDrag/Autonomous Controller /Take-off switch ==
  Auto Take-off out : Inport
  Auto Enroute out : Inport  Port=2
  Bus Creator : BusCreator  Inputs='roll','pitch','thrust','yaw','noseWheel','status'
  Bus Selector : BusSelector  OutputSignals=roll,pitch,thrust,yaw,status
  Bus Selector1 : BusSelector  OutputSignals=status,roll,pitch,thrust,yaw,noseWheel
  pitch switch : Switch  Criteria=u2 > Threshold
  roll switch : Switch  Criteria=u2 > Threshold
  thrust switch : Switch  Criteria=u2 > Threshold
  yaw switch : Switch  Criteria=u2 > Threshold
  Enroute out : Outport
  wires:
  Bus Selector1/2 -> roll switch/3  "<roll>"
  roll switch/1 -> Bus Creator/1  "roll"
  Bus Selector1/3 -> pitch switch/3  "<pitch>"
  pitch switch/1 -> Bus Creator/2  "pitch"
  Bus Selector1/4 -> thrust switch/3  "<thrust>"
  thrust switch/1 -> Bus Creator/3  "thrust"
  Bus Selector1/1 -> yaw switch/2, thrust switch/2, pitch switch/2, roll switch/2  "<status>"
  Bus Selector1/5 -> yaw switch/3  "<yaw>"
  yaw switch/1 -> Bus Creator/4  "yaw"
  Bus Selector/1 -> roll switch/1  "<roll>"
  Bus Selector/2 -> pitch switch/1  "<pitch>"
  Bus Selector/3 -> thrust switch/1  "<thrust>"
  Bus Selector/4 -> yaw switch/1  "<yaw>"
  Auto Enroute out/1 -> Bus Selector/1
  Auto Take-off out/1 -> Bus Selector1/1
  Bus Selector1/6 -> Bus Creator/5  "<noseWheel>"
  Bus Creator/1 -> Enroute out/1
  Bus Selector/5 -> Bus Creator/6  "<status>"

== system TestDrag/Get data from XPlane/3-mission time ==
  In2 : Inport
  Memory2 : Memory
  Switch2 : Switch  Criteria=u2 ~= 0
  Out1 : Outport
  wires:
  Memory2/1 -> Switch2/3, Out1/1
  Switch2/1 -> Memory2/1
  In2/1 -> Switch2/1, Switch2/2

== system TestDrag/Get data from XPlane/continuous ==
  In2 : Inport
  Memory2 : Memory
  Switch2 : Switch  Criteria=u2 ~= 0
  Out1 : Outport
  wires:
  Memory2/1 -> Switch2/3, Out1/1
  Switch2/1 -> Memory2/1
  In2/1 -> Switch2/1, Switch2/2

== system TestDrag/Get data from XPlane/continuous1 ==
  In2 : Inport
  Memory2 : Memory
  Switch2 : Switch  Criteria=u2 ~= 0
  Out1 : Outport
  wires:
  Memory2/1 -> Switch2/3, Out1/1
  Switch2/1 -> Memory2/1
  In2/1 -> Switch2/1, Switch2/2

== system TestDrag/Get data from XPlane/continuous10 ==
  In2 : Inport
  Memory2 : Memory
  Switch2 : Switch  Criteria=u2 ~= 0
  Out1 : Outport
  wires:
  Memory2/1 -> Switch2/3, Out1/1
  Switch2/1 -> Memory2/1
  In2/1 -> Switch2/1, Switch2/2

== system TestDrag/Get data from XPlane/continuous11 ==
  In2 : Inport
  Memory2 : Memory
  Switch2 : Switch  Criteria=u2 ~= 0
  Out1 : Outport
  wires:
  Memory2/1 -> Switch2/3, Out1/1
  Switch2/1 -> Memory2/1
  In2/1 -> Switch2/1, Switch2/2

== system TestDrag/Get data from XPlane/continuous12 ==
  In2 : Inport
  Memory2 : Memory
  Switch2 : Switch  Criteria=u2 ~= 0
  Out1 : Outport
  wires:
  Memory2/1 -> Switch2/3, Out1/1
  Switch2/1 -> Memory2/1
  In2/1 -> Switch2/1, Switch2/2

== system TestDrag/Get data from XPlane/continuous13 ==
  In2 : Inport
  Memory2 : Memory
  Switch2 : Switch  Criteria=u2 ~= 0
  Out1 : Outport
  wires:
  Memory2/1 -> Switch2/3, Out1/1
  Switch2/1 -> Memory2/1
  In2/1 -> Switch2/1, Switch2/2

== system TestDrag/Get data from XPlane/continuous14 ==
  In2 : Inport
  Memory2 : Memory
  Switch2 : Switch  Criteria=u2 ~= 0
  Out1 : Outport
  wires:
  Memory2/1 -> Switch2/3, Out1/1
  Switch2/1 -> Memory2/1
  In2/1 -> Switch2/1, Switch2/2

== system TestDrag/Get data from XPlane/continuous15 ==
  In2 : Inport
  Memory2 : Memory
  Switch2 : Switch  Criteria=u2 ~= 0
  Out1 : Outport
  wires:
  Memory2/1 -> Switch2/3, Out1/1
  Switch2/1 -> Memory2/1
  In2/1 -> Switch2/1, Switch2/2

== system TestDrag/Get data from XPlane/continuous16 ==
  In2 : Inport
  Memory2 : Memory
  Switch2 : Switch  Criteria=u2 ~= 0
  Out1 : Outport
  wires:
  Memory2/1 -> Switch2/3, Out1/1
  Switch2/1 -> Memory2/1
  In2/1 -> Switch2/1, Switch2/2

== system TestDrag/Get data from XPlane/continuous17 ==
  In2 : Inport
  Memory2 : Memory
  Switch2 : Switch  Criteria=u2 ~= 0
  Out1 : Outport
  wires:
  Memory2/1 -> Switch2/3, Out1/1
  Switch2/1 -> Memory2/1
  In2/1 -> Switch2/1, Switch2/2

== system TestDrag/Get data from XPlane/continuous18 ==
  In2 : Inport
  Memory2 : Memory
  Switch2 : Switch  Criteria=u2 ~= 0
  Out1 : Outport
  wires:
  Memory2/1 -> Switch2/3, Out1/1
  Switch2/1 -> Memory2/1
  In2/1 -> Switch2/1, Switch2/2

== system TestDrag/Get data from XPlane/continuous2 ==
  In2 : Inport
  Memory2 : Memory
  Switch2 : Switch  Criteria=u2 ~= 0
  Out1 : Outport
  wires:
  Memory2/1 -> Switch2/3, Out1/1
  Switch2/1 -> Memory2/1
  In2/1 -> Switch2/1, Switch2/2

== system TestDrag/Get data from XPlane/continuous3 ==
  In2 : Inport
  Memory2 : Memory
  Switch2 : Switch  Criteria=u2 ~= 0
  Out1 : Outport
  wires:
  Memory2/1 -> Switch2/3, Out1/1
  Switch2/1 -> Memory2/1
  In2/1 -> Switch2/1, Switch2/2

== system TestDrag/Get data from XPlane/continuous4 ==
  In2 : Inport
  Memory2 : Memory
  Switch2 : Switch  Criteria=u2 ~= 0
  Out1 : Outport
  wires:
  Memory2/1 -> Switch2/3, Out1/1
  Switch2/1 -> Memory2/1
  In2/1 -> Switch2/1, Switch2/2

== system TestDrag/Get data from XPlane/continuous5 ==
  In2 : Inport
  Memory2 : Memory
  Switch2 : Switch  Criteria=u2 ~= 0
  Out1 : Outport
  wires:
  Memory2/1 -> Switch2/3, Out1/1
  Switch2/1 -> Memory2/1
  In2/1 -> Switch2/1, Switch2/2

== system TestDrag/Get data from XPlane/continuous6 ==
  In2 : Inport
  Memory2 : Memory
  Switch2 : Switch  Criteria=u2 ~= 0
  Out1 : Outport
  wires:
  Memory2/1 -> Switch2/3, Out1/1
  Switch2/1 -> Memory2/1
  In2/1 -> Switch2/1, Switch2/2

== system TestDrag/Get data from XPlane/continuous7 ==
  In2 : Inport
  Memory2 : Memory
  Switch2 : Switch  Criteria=u2 ~= 0
  Out1 : Outport
  wires:
  Memory2/1 -> Switch2/3, Out1/1
  Switch2/1 -> Memory2/1
  In2/1 -> Switch2/1, Switch2/2

== system TestDrag/Get data from XPlane/continuous8 ==
  In2 : Inport
  Memory2 : Memory
  Switch2 : Switch  Criteria=u2 ~= 0
  Out1 : Outport
  wires:
  Memory2/1 -> Switch2/3, Out1/1
  Switch2/1 -> Memory2/1
  In2/1 -> Switch2/1, Switch2/2

== system TestDrag/Get data from XPlane/continuous9 ==
  In2 : Inport
  Memory2 : Memory
  Switch2 : Switch  Criteria=u2 ~= 0
  Out1 : Outport
  wires:
  Memory2/1 -> Switch2/3, Out1/1
  Switch2/1 -> Memory2/1
  In2/1 -> Switch2/1, Switch2/2

== system TestDrag/Autonomous Controller /Attitude Controller/normalize ==
  In : Inport
  Minus Offset : Constant  Value=-360
  Offset : Constant  Value=360
  Sum1 : Sum  Inputs=|++
  Sum7 : Sum  Inputs=|++
  Switch : Switch  Criteria=u2 > Threshold  Threshold=-180
  Switch1 : Switch  Criteria=u2 > Threshold  Threshold=180
  Out : Outport
  wires:
  Offset/1 -> Sum7/2
  Sum7/1 -> Switch/3
  In/1 -> Switch/2, Switch/1, Sum1/2, Switch1/2, Sum7/1
  Sum1/1 -> Switch1/1
  Minus Offset/1 -> Sum1/1
  Switch/1 -> Switch1/3
  Switch1/1 -> Out/1

== system TestDrag/Autonomous Controller /Auto Landing/Desired Altitude ==
  Alt : Inport
  1-D Lookup Table : Lookup_n-D  NumberOfTableDimensions=1  BreakpointsForDimension1=[10,13,17,23,30,40,50]  Table=[0.5,0.4,0.3,0.2,0.1,0,-0.1]  InternalRulePriority=Speed  RndMeth=Simplest  InputSameDT=on
  pitch : Outport
  wires:
  Alt/1 -> 1-D Lookup Table/1
  1-D Lookup Table/1 -> pitch/1

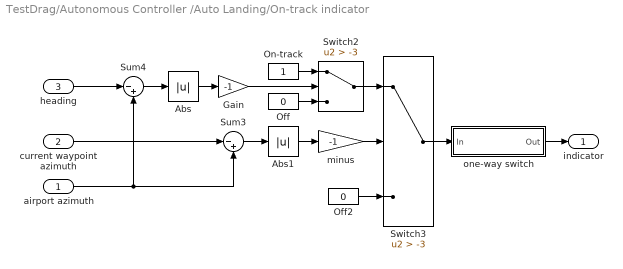
== system TestDrag/Autonomous Controller /Auto Landing/On-track indicator ==
  airport azimuth : Inport
  current waypoint azimuth : Inport  Port=2
  heading : Inport  Port=3
  Abs : Abs
  Abs1 : Abs
  Gain : Gain  Gain=-1
  Off : Constant  Value=0
  Off2 : Constant  Value=0
  On-track : Constant
  Sum3 : Sum  Inputs=|-+
  Sum4 : Sum  Inputs=|-+
  Switch2 : Switch  Criteria=u2 > Threshold  Threshold=-3
  Switch3 : Switch  Criteria=u2 > Threshold  Threshold=-3
  minus : Gain  Gain=-1
  "one-way switch " : Subsystem
  indicator : Outport
  wires:
  Sum4/1 -> Abs/1
  On-track/1 -> Switch2/1
  Abs/1 -> Gain/1
  minus/1 -> Switch3/2
  current waypoint azimuth/1 -> Sum3/1
  airport azimuth/1 -> Sum3/2, Sum4/2
  Gain/1 -> Switch2/2
  "one-way switch "/1(Out) -> indicator/1
  Switch3/1 -> "one-way switch "/1(In)
  Off/1 -> Switch2/3
  Switch2/1 -> Switch3/1
  Abs1/1 -> minus/1
  Sum3/1 -> Abs1/1
  Off2/1 -> Switch3/3
  heading/1 -> Sum4/1

== system TestDrag/Autonomous Controller /Auto Landing/normalize ==
  In : Inport
  Minus Offset : Constant  Value=-360
  Offset : Constant  Value=360
  Sum1 : Sum  Inputs=|++
  Sum7 : Sum  Inputs=|++
  Switch : Switch  Criteria=u2 > Threshold  Threshold=-180
  Switch1 : Switch  Criteria=u2 > Threshold  Threshold=180
  Out : Outport
  wires:
  Offset/1 -> Sum7/2
  Sum7/1 -> Switch/3
  In/1 -> Switch/2, Switch/1, Sum1/2, Switch1/2, Sum7/1
  Sum1/1 -> Switch1/1
  Minus Offset/1 -> Sum1/1
  Switch/1 -> Switch1/3
  Switch1/1 -> Out/1

== system TestDrag/Autonomous Controller /Auto Landing/normalize1 ==
  In : Inport
  Constant : Constant  Value=360
  Sum7 : Sum  Inputs=|++
  Switch : Switch  Criteria=u2 > Threshold  Threshold=-180
  Out : Outport
  wires:
  Switch/1 -> Out/1
  Constant/1 -> Sum7/2
  Sum7/1 -> Switch/3
  In/1 -> Switch/2, Switch/1, Sum7/1

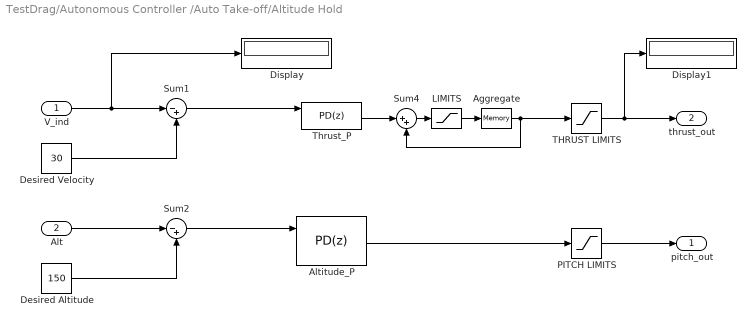
== system TestDrag/Autonomous Controller /Auto Take-off/Altitude Hold ==
  V_ind : Inport
  Alt : Inport  Port=2
  Aggregate : Memory  X0=1  InheritSampleTime=on  LinearizeMemory=on  LinearizeAsDelay=on
  Altitude_P : simulink/Continuous/PID Controller  Controller=PD  TimeDomain=Discrete-time  SampleTime=0.02  IntegratorMethod=Forward Euler  FilterMethod=Forward Euler  Form=Parallel  UseFilter=off  ControllerParametersSource=internal  P=0.12  I=0.0003  D=0.0024  N=20  InitialConditionSource=internal  InitialConditionForIntegrator=0  InitialConditionForFilter=0  ExternalReset=either  LimitOutput=on  UpperSaturationLimit=1  LowerSaturationLimit=-1  LinearizeAsGain=on  AntiWindupMode=none  Kb=1  TrackingMode=off  Kt=1  PParamMin=[]  PParamMax=[]  IParamMin=[]  IParamMax=[]  DParamMin=[]  DParamMax=[]  NParamMin=[]  NParamMax=[]  KbParamMin=[]  KbParamMax=[]  KtParamMin=[]  KtParamMax=[]  POutMin=[]  POutMax=[]  IOutMin=[]  IOutMax=[]  DOutMin=[]  DOutMax=[]  NOutMin=[]  NOutMax=[]  KbOutMin=[]  KbOutMax=[]  KtOutMin=[]  KtOutMax=[]  IntegratorOutMin=[]  IntegratorOutMax=[]  FilterOutMin=[]  FilterOutMax=[]  SumOutMin=[]  SumOutMax=[]  SumI1OutMin=[]  SumI1OutMax=[]  SumI2OutMin=[]  SumI2OutMax=[]  SumI3OutMin=[]  SumI3OutMax=[]  SumDOutMin=[]  SumDOutMax=[]  SaturationOutMin=[]  SaturationOutMax=[]  IntegratorContinuousStateAttributes=''  IntegratorStateMustResolveToSignalObject=off  IntegratorRTWStateStorageClass=Auto  FilterContinuousStateAttributes=''  FilterStateMustResolveToSignalObject=off  FilterRTWStateStorageClass=Auto  DifferentiatorICPrevScaledInput=0  DifferentiatorOutMin=[]  DifferentiatorOutMax=[]
  Desired Altitude : Constant  Value=150  OutDataTypeStr=single
  Desired Velocity : Constant  Value=30  OutDataTypeStr=single
  Display : Display
  Display1 : Display
  LIMITS : Saturate  UpperLimit=1  LowerLimit=0
  PITCH LIMITS : Saturate  UpperLimit=0.4  LowerLimit=-0.4
  Sum1 : Sum  Inputs=|-+
  Sum2 : Sum  Inputs=|-+
  Sum4 : Sum  Inputs=|++
  THRUST LIMITS : Saturate  UpperLimit=1  LowerLimit=0
  Thrust_P : simulink/Continuous/PID Controller  Controller=PD  TimeDomain=Discrete-time  SampleTime=0.02  IntegratorMethod=Forward Euler  FilterMethod=Forward Euler  Form=Parallel  UseFilter=off  ControllerParametersSource=internal  P=0.0005  I=0.0000000001  D=0.003  N=20  InitialConditionSource=internal  InitialConditionForIntegrator=0  InitialConditionForFilter=0  ExternalReset=either  LimitOutput=on  UpperSaturationLimit=1  LowerSaturationLimit=-1  LinearizeAsGain=on  AntiWindupMode=none  Kb=1  TrackingMode=off  Kt=1  PParamMin=[]  PParamMax=[]  IParamMin=[]  IParamMax=[]  DParamMin=[]  DParamMax=[]  NParamMin=[]  NParamMax=[]  KbParamMin=[]  KbParamMax=[]  KtParamMin=[]  KtParamMax=[]  POutMin=[]  POutMax=[]  IOutMin=[]  IOutMax=[]  DOutMin=[]  DOutMax=[]  NOutMin=[]  NOutMax=[]  KbOutMin=[]  KbOutMax=[]  KtOutMin=[]  KtOutMax=[]  IntegratorOutMin=[]  IntegratorOutMax=[]  FilterOutMin=[]  FilterOutMax=[]  SumOutMin=[]  SumOutMax=[]  SumI1OutMin=[]  SumI1OutMax=[]  SumI2OutMin=[]  SumI2OutMax=[]  SumI3OutMin=[]  SumI3OutMax=[]  SumDOutMin=[]  SumDOutMax=[]  SaturationOutMin=[]  SaturationOutMax=[]  IntegratorContinuousStateAttributes=''  IntegratorStateMustResolveToSignalObject=off  IntegratorRTWStateStorageClass=Auto  FilterContinuousStateAttributes=''  FilterStateMustResolveToSignalObject=off  FilterRTWStateStorageClass=Auto  DifferentiatorICPrevScaledInput=0  DifferentiatorOutMin=[]  DifferentiatorOutMax=[]
  pitch_out : Outport
  thrust_out : Outport  Port=2
  wires:
  PITCH LIMITS/1 -> pitch_out/1
  Sum2/1 -> Altitude_P/1
  Desired Altitude/1 -> Sum2/2
  Altitude_P/1 -> PITCH LIMITS/1
  Sum1/1 -> Thrust_P/1
  Desired Velocity/1 -> Sum1/2
  Sum4/1 -> LIMITS/1
  Thrust_P/1 -> Sum4/1
  Alt/1 -> Sum2/1
  V_ind/1 -> Display/1, Sum1/1
  Aggregate/1 -> Sum4/2, THRUST LIMITS/1
  THRUST LIMITS/1 -> Display1/1, thrust_out/1
  LIMITS/1 -> Aggregate/1

== system TestDrag/Autonomous Controller /Auto Take-off/Altitude Indicator ==
  Altitude : Inport
  Saturated : Constant  OutDataTypeStr=single
  Unsaturated : Constant  Value=0  OutDataTypeStr=single
  "one-way switch " : Subsystem
  switch : Switch  Threshold=30
  Indicator : Outport
  wires:
  Saturated/1 -> switch/1
  Unsaturated/1 -> switch/3
  Altitude/1 -> switch/2
  "one-way switch "/1(Out) -> Indicator/1
  switch/1 -> "one-way switch "/1(In)

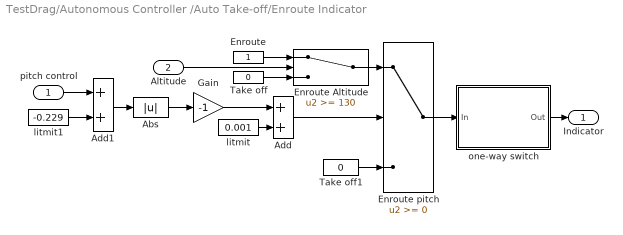
== system TestDrag/Autonomous Controller /Auto Take-off/Enroute Indicator ==
  pitch control : Inport
  Altitude : Inport  Port=2
  Abs : Abs
  Add : Sum
  Add1 : Sum
  Enroute : Constant  OutDataTypeStr=single
  Enroute Altitude : Switch  Threshold=130
  Enroute pitch : Switch
  Gain : Gain  Gain=-1
  Take off : Constant  Value=0  OutDataTypeStr=single
  Take off1 : Constant  Value=0  OutDataTypeStr=single
  litmit : Constant  Value=0.001
  litmit1 : Constant  Value=-0.229
  "one-way switch " : Subsystem
  Indicator : Outport
  wires:
  Enroute/1 -> Enroute Altitude/1
  Take off/1 -> Enroute Altitude/3
  Altitude/1 -> Enroute Altitude/2
  "one-way switch "/1(Out) -> Indicator/1
  Abs/1 -> Gain/1
  litmit/1 -> Add/2
  Add/1 -> Enroute pitch/2
  Gain/1 -> Add/1
  Enroute Altitude/1 -> Enroute pitch/1
  Take off1/1 -> Enroute pitch/3
  Enroute pitch/1 -> "one-way switch "/1(In)
  pitch control/1 -> Add1/1
  litmit1/1 -> Add1/2
  Add1/1 -> Abs/1

== system TestDrag/Autonomous Controller /Auto Take-off/normalize ==
  In : Inport
  Minus Offset : Constant  Value=-360
  Offset : Constant  Value=360
  Sum1 : Sum  Inputs=|++
  Sum7 : Sum  Inputs=|++
  Switch : Switch  Criteria=u2 > Threshold  Threshold=-180
  Switch1 : Switch  Criteria=u2 > Threshold  Threshold=180
  Out : Outport
  wires:
  Offset/1 -> Sum7/2
  Sum7/1 -> Switch/3
  In/1 -> Switch/2, Switch/1, Sum1/2, Switch1/2, Sum7/1
  Sum1/1 -> Switch1/1
  Minus Offset/1 -> Sum1/1
  Switch/1 -> Switch1/3
  Switch1/1 -> Out/1

== system TestDrag/Autonomous Controller /Auto enroute/Altitude Hold ==
  Desired Velocity : Constant  Value=0  OutDataTypeStr=single
  Desired Velocity1 : Constant  Value=0.12  OutDataTypeStr=single
  PITCH LIMITS : Saturate  UpperLimit=1  LowerLimit=-1
  THRUST LIMITS : Saturate  UpperLimit=1  LowerLimit=0
  pitch_out : Outport
  thrust_out : Outport  Port=2
  wires:
  PITCH LIMITS/1 -> pitch_out/1
  THRUST LIMITS/1 -> thrust_out/1
  Desired Velocity/1 -> THRUST LIMITS/1
  Desired Velocity1/1 -> PITCH LIMITS/1

== system TestDrag/Autonomous Controller /Auto Landing/On-track indicator/one-way switch  ==
  In : Inport
  Memory4 : Memory  InheritSampleTime=on
  Switch8 : Switch  Criteria=u2 > Threshold
  Out : Outport
  wires:
  Memory4/1 -> Out/1, Switch8/3
  Switch8/1 -> Memory4/1
  In/1 -> Switch8/1, Switch8/2

== system TestDrag/Autonomous Controller /Auto Take-off/Altitude Indicator/one-way switch  ==
  In : Inport
  Memory4 : Memory  InheritSampleTime=on
  Switch8 : Switch  Criteria=u2 > Threshold
  Out : Outport
  wires:
  Memory4/1 -> Out/1, Switch8/3
  Switch8/1 -> Memory4/1
  In/1 -> Switch8/1, Switch8/2

== system TestDrag/Autonomous Controller /Auto Take-off/Enroute Indicator/one-way switch  ==
  In : Inport
  Memory4 : Memory  InheritSampleTime=on
  Switch8 : Switch  Criteria=u2 > Threshold
  Out : Outport
  wires:
  Memory4/1 -> Out/1, Switch8/3
  Switch8/1 -> Memory4/1
  In/1 -> Switch8/1, Switch8/2

== matlab function TestDrag/Send to XPlane10/'DATA0' ==
  data: y output
function y = fcn()
%#codegen
%y=uint8(zeros(1,77));
y = uint8('DATA0');

== matlab function TestDrag/Get data from XPlane/MATLAB Function ==
  data: u input; Data output single size=[75 8]; msgLen input
function Data  = fcn(u,msgLen)
%#codegen
%coder.extrinsic('clear')
dataLen=msgLen-5;
Npackets=dataLen/36;

% initialize data matrix
% rows: packets of data; columns: data values, first column is the data
% index
maxNPackets=75;
Nvalues=8;% number of values in each packet
Data=single(zeros(maxNPackets,Nvalues));

Bytecounter=6; % start after the 5th byte

for i=1:msgLen
    
    if char(u(i))=='D' && char(u(i+1))=='A'
        %loop over each packet
        for j=1:Npackets
                indx=typecast(u(Bytecounter:Bytecounter+3),'uint32');% packet index
                %Data(indx,1)=single(indx); % packet index
                Bytecounter=Bytecounter+4; % go to the next 4 bytes
                Data(indx,1)=typecast(u(Bytecounter:Bytecounter+3),'single'); % 1st value
                Bytecounter=Bytecounter+4; % go to the next 4 bytes
                Data(indx,2)=typecast(u(Bytecounter:Bytecounter+3),'single'); % 2nd value
                Bytecounter=Bytecounter+4; % go to the next 4 bytes
                Data(indx,3)=typecast(u(Bytecounter:Bytecounter+3),'single'); % 3rd value
                Bytecounter=Bytecounter+4; % go to the next 4 bytes
                Data(indx,4)=typecast(u(Bytecounter:Bytecounter+3),'single'); % 4th value
                Bytecounter=Bytecounter+4; % go to the next 4 bytes
                Data(indx,5)=typecast(u(Bytecounter:Bytecounter+3),'single'); % 5th value
                Bytecounter=Bytecounter+4; % go to the next 4 bytes
                Data(indx,6)=typecast(u(Bytecounter:Bytecounter+3),'single'); % 6th value
                Bytecounter=Bytecounter+4; % go to the next 4 bytes
                Data(indx,7)=typecast(u(Bytecounter:Bytecounter+3),'single'); % 7th value
                Bytecounter=Bytecounter+4; % go to the next 4 bytes
                Data(indx,8)=typecast(u(Bytecounter:Bytecounter+3),'single'); % 8th value
                Bytecounter=Bytecounter+4;% go to the next packet index 
        end
        break
    end
end
%clear Data

== matlab function TestDrag/MATLAB Function1 ==
  data: AirportCoordinates output
function AirportCoordinates = getWP()
AirportCoordinates = [21.219041824340820 105.8135528564453 50; 21.225227355957030 105.7927398681641 50];
% AirportCoordinates = [21.219041824340820 105.8135528564453 50; 21.221620559692383 1.058050003051758e+02 50; 21.225227355957030 105.7927398681641 50];
% WPdataTable = [21.215 105.798 50; 21.219041824340820 105.8135528564453 50; 21.225227355957030 105.7927398681641 50];
% 21.220420837402344 1.058090286254883e+02;
% 21.221620559692383 1.058050003051758e+02;

== matlab function TestDrag/MATLAB Function2 ==
  data: WPdataTable output
function WPdataTable = getWP()
WPdataTable = [21.215 105.798 50; 21.219041824340820 105.8135528564453 50];
% WPdataTable = [21.215 105.798 50; 21.219041824340820 105.8135528564453 50; 21.225227355957030 105.7927398681641 50];
% 21.220420837402344 1.058090286254883e+02;
% 21.221620559692383 1.058050003051758e+02;

== matlab function TestDrag/Autonomous Controller /Auto Landing/MATLAB Function2 ==
  data: currentPosition input; WP input; ref_azimuth output; curr_azimuth output
function [ref_azimuth, curr_azimuth] = currentWP(currentPosition, WP)
%=============================Intitialization==============================
persistent initialize curr_buff;
    
if isempty(initialize)
    if isempty(curr_buff)        
        curr_buff = coder.nullcopy(zeros(1));
        ref_azimuth = coder.nullcopy(zeros(1));
    end        
    initialize = 1;     
end
%Declare patch as extrinsic
coder.extrinsic('azimuth'); 
curr_buff = azimuth(currentPosition(1),currentPosition(2),WP(2,1),WP(2,2));
ref_azimuth = azimuth(WP(1,1),WP(1,2),WP(2,1),WP(2,2));
curr_azimuth = curr_buff;
